simulink model "iir_10th_order"  (R2020b)
settings: Solver=FixedStepDiscrete  StartTime=0.0  StopTime=stopTime  FixedStep=2.0833333333333333e-05  RelTol=1e-3
settings Model: Creator=Ross  LastModifiedBy=conno
settings DataIOCC: SaveOutput=off  SaveTime=off  ReturnWorkspaceOutputs=off
settings OptimizationCC: BlockReduction=off  ConditionallyExecuteInputs=off  DefaultParameterBehavior=Inlined
settings DebuggingCC: ReadBeforeWriteMsg=DisableAll  WriteAfterWriteMsg=DisableAll  WriteAfterReadMsg=DisableAll  AlgebraicLoopMsg=error  MultiTaskDSMMsg=none  SingleTaskRateTransMsg=error  PregeneratedLibrarySubsystemCodeDiagnostic=none  ArithmeticOperatorsInVariantConditions=warning
settings HardwareCC: ProdBitPerPointer=32  ProdBitPerSizeT=32  ProdBitPerPtrDiffT=32  ProdLargestAtomicFloat=None  ProdIntDivRoundTo=Undefined  ProdEndianess=Unspecified  ProdWordSize=32  ProdHWDeviceType=ASIC/FPGA->ASIC/FPGA  TargetBitPerPointer=64  TargetBitPerSizeT=64  TargetBitPerPtrDiffT=64  TargetLongLongMode=on  TargetIntDivRoundTo=Zero  TargetEndianess=LittleEndian  TargetWordSize=64  TargetHWDeviceType=Custom Processor->MATLAB Host Computer  ProdEqTarget=off
settings ModelReferenceCC: UpdateModelReferenceTargets=IfOutOfDate
settings SFSimCC: SFSimEcho=off  SimUseLocalCustomCode=off  CustomCodeUndefinedFunction=UseInterfaceOnly
settings RTWCC: RTWUseLocalCustomCode=off

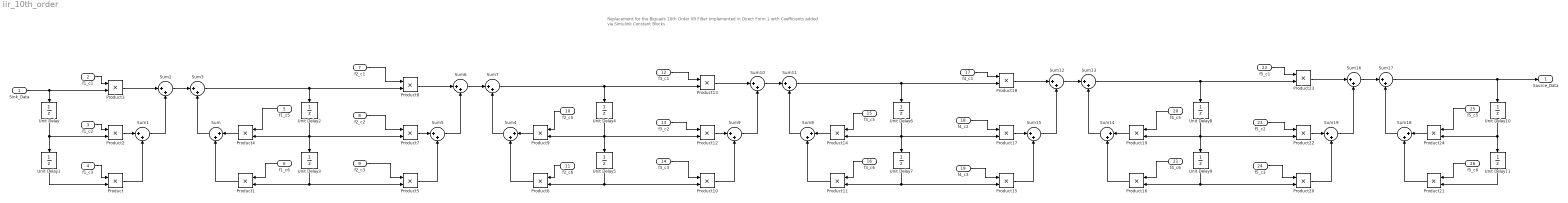
== system iir_10th_order ==
  note: Replacement for the Biquads
      | 10th Order IIR Filter Implemented in Direct Form 1 with Coefficients added via Simulink Constant Blocks
  Sink_Data : Inport  OutDataTypeStr=single  PortDimensions=1  SampleTime=[2.0833333333333333e-05,0]
  f1_c1 : Inport  Port=2  OutDataTypeStr=single  PortDimensions=1  SampleTime=[2.0833333333333333e-05,0]
  f1_c2 : Inport  Port=3  OutDataTypeStr=single  PortDimensions=1  SampleTime=[2.0833333333333333e-05,0]
  f1_c3 : Inport  Port=4  OutDataTypeStr=single  PortDimensions=1  SampleTime=[2.0833333333333333e-05,0]
  f1_c5 : Inport  Port=5  OutDataTypeStr=single  PortDimensions=1  SampleTime=[2.0833333333333333e-05,0]
  f1_c6 : Inport  Port=6  OutDataTypeStr=single  PortDimensions=1  SampleTime=[2.0833333333333333e-05,0]
  f2_c1 : Inport  Port=7  OutDataTypeStr=single  PortDimensions=1  SampleTime=[2.0833333333333333e-05,0]
  f2_c2 : Inport  Port=8  OutDataTypeStr=single  PortDimensions=1  SampleTime=[2.0833333333333333e-05,0]
  f2_c3 : Inport  Port=9  OutDataTypeStr=single  PortDimensions=1  SampleTime=[2.0833333333333333e-05,0]
  f2_c5 : Inport  Port=10  OutDataTypeStr=single  PortDimensions=1  SampleTime=[2.0833333333333333e-05,0]
  f2_c6 : Inport  Port=11  OutDataTypeStr=single  PortDimensions=1  SampleTime=[2.0833333333333333e-05,0]
  f3_c1 : Inport  Port=12  OutDataTypeStr=single  PortDimensions=1  SampleTime=[2.0833333333333333e-05,0]
  f3_c2 : Inport  Port=13  OutDataTypeStr=single  PortDimensions=1  SampleTime=[2.0833333333333333e-05,0]
  f3_c3 : Inport  Port=14  OutDataTypeStr=single  PortDimensions=1  SampleTime=[2.0833333333333333e-05,0]
  f3_c5 : Inport  Port=15  OutDataTypeStr=single  PortDimensions=1  SampleTime=[2.0833333333333333e-05,0]
  f3_c6 : Inport  Port=16  OutDataTypeStr=single  PortDimensions=1  SampleTime=[2.0833333333333333e-05,0]
  f4_c1 : Inport  Port=17  OutDataTypeStr=single  PortDimensions=1  SampleTime=[2.0833333333333333e-05,0]
  f4_c2 : Inport  Port=18  OutDataTypeStr=single  PortDimensions=1  SampleTime=[2.0833333333333333e-05,0]
  f4_c3 : Inport  Port=19  OutDataTypeStr=single  PortDimensions=1  SampleTime=[2.0833333333333333e-05,0]
  f4_c5 : Inport  Port=20  OutDataTypeStr=single  PortDimensions=1  SampleTime=[2.0833333333333333e-05,0]
  f4_c6 : Inport  Port=21  OutDataTypeStr=single  PortDimensions=1  SampleTime=[2.0833333333333333e-05,0]
  f5_c1 : Inport  Port=22  OutDataTypeStr=single  PortDimensions=1  SampleTime=[2.0833333333333333e-05,0]
  f5_c2 : Inport  Port=23  OutDataTypeStr=single  PortDimensions=1  SampleTime=[2.0833333333333333e-05,0]
  f5_c3 : Inport  Port=24  OutDataTypeStr=single  PortDimensions=1  SampleTime=[2.0833333333333333e-05,0]
  f5_c5 : Inport  Port=25  OutDataTypeStr=single  PortDimensions=1  SampleTime=[2.0833333333333333e-05,0]
  f5_c6 : Inport  Port=26  OutDataTypeStr=single  PortDimensions=1  SampleTime=[2.0833333333333333e-05,0]
  Product{,1..24} (25 alike) : Product
  Sum{,1..19} (20 alike) : Sum  Inputs=|++
  Unit Delay{,1..11} (12 alike) : UnitDelay  SampleTime=-1  HasFrameUpgradeWarning=on
  Source_Data : Outport  OutDataTypeStr=single  PortDimensions=1  SampleTime=[2.0833333333333333e-05,0]
  wires:
  Sum12/1 -> Sum13/1
  Product19/1 -> Sum14/1
  Product1/1 -> Sum/2
  Product24/1 -> Sum18/1
  f5_c1/1 -> Product23/1
  Product21/1 -> Sum18/2
  f1_c1/1 -> Product3/1
  f2_c1/1 -> Product8/1
  Sink_Data/1 -> Product3/2, Unit Delay/1
  Unit Delay9/1 -> Product16/2, Product20/2
  Product8/1 -> Sum6/1
  Product12/1 -> Sum9/1
  f4_c3/1 -> Product15/1
  Sum18/1 -> Sum17/2
  f5_c2/1 -> Product22/1
  Product11/1 -> Sum8/2
  Product15/1 -> Sum15/2
  Product22/1 -> Sum19/1
  Product7/1 -> Sum5/1
  Unit Delay6/1 -> Product14/2, Product17/2, Unit Delay7/1
  Product16/1 -> Sum14/2
  Sum13/1 -> Unit Delay8/1, Product23/2
  Sum7/1 -> Unit Delay4/1, Product13/2
  Unit Delay1/1 -> Product/2
  Product6/1 -> Sum4/2
  Unit Delay7/1 -> Product11/2, Product15/2
  Sum9/1 -> Sum10/2
  Unit Delay2/1 -> Product4/2, Product7/2, Unit Delay3/1
  Sum8/1 -> Sum11/2
  Unit Delay8/1 -> Unit Delay9/1, Product19/2, Product22/2
  Sum10/1 -> Sum11/1
  Product14/1 -> Sum8/1
  Unit Delay5/1 -> Product6/2, Product10/2
  Unit Delay10/1 -> Product24/2, Unit Delay11/1
  Sum/1 -> Sum3/2
  Sum11/1 -> Unit Delay6/1, Product18/2
  Product18/1 -> Sum12/1
  f3_c2/1 -> Product12/1
  Sum16/1 -> Sum17/1
  f2_c3/1 -> Product5/1
  f4_c2/1 -> Product17/1
  f1_c2/1 -> Product2/1
  Product20/1 -> Sum19/2
  Product3/1 -> Sum2/1
  Product23/1 -> Sum16/1
  Sum3/1 -> Unit Delay2/1, Product8/2
  Product9/1 -> Sum4/1
  f3_c3/1 -> Product10/1
  Sum19/1 -> Sum16/2
  Unit Delay/1 -> Unit Delay1/1, Product2/2
  Unit Delay4/1 -> Product9/2, Product12/2, Unit Delay5/1
  Product10/1 -> Sum9/2
  Sum15/1 -> Sum12/2
  Product13/1 -> Sum10/1
  Sum17/1 -> Unit Delay10/1, Source_Data/1
  Unit Delay3/1 -> Product1/2, Product5/2
  f3_c1/1 -> Product13/1
  Product17/1 -> Sum15/1
  Product4/1 -> Sum/1
  f4_c1/1 -> Product18/1
  Sum4/1 -> Sum7/2
  f1_c3/1 -> Product/1
  f1_c5/1 -> Product4/1
  Unit Delay11/1 -> Product21/2
  Product2/1 -> Sum1/1
  Product5/1 -> Sum5/2
  Sum14/1 -> Sum13/2
  f2_c2/1 -> Product7/1
  Sum2/1 -> Sum3/1
  Sum6/1 -> Sum7/1
  Sum1/1 -> Sum2/2
  Product/1 -> Sum1/2
  Sum5/1 -> Sum6/2
  f1_c6/1 -> Product1/1
  f2_c6/1 -> Product6/1
  f2_c5/1 -> Product9/1
  f3_c5/1 -> Product14/1
  f3_c6/1 -> Product11/1
  f4_c5/1 -> Product19/1
  f4_c6/1 -> Product16/1
  f5_c3/1 -> Product20/1
  f5_c5/1 -> Product24/1
  f5_c6/1 -> Product21/1
